simulink model "HW2_FSR_ES4"  (R2023b)
settings: Solver=FixedStepAuto  StartTime=0.0  StopTime=T  FixedStep=Ts  RelTol=1e-5
values from neighbouring files (symbols this model uses):
  k1 = 1    [HW2_FSR_ES4_Script.m]
  k2 = 2    [HW2_FSR_ES4_Script.m]
  k3 = 1    [HW2_FSR_ES4_Script.m]
  q_i = [10 1 pi\4]'    [HW2_FSR_ES4_Script.m]
  Ts = 0.01    [HW2_FSR_ES4_Script.m]
libraries: robotmobilelib x1
settings Model: Creator=emman  LastModifiedBy=emman

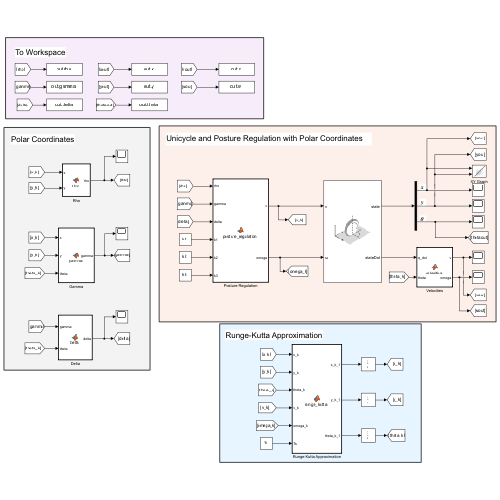
[thumbnail: Simulink's stored preview of the top-level diagram]
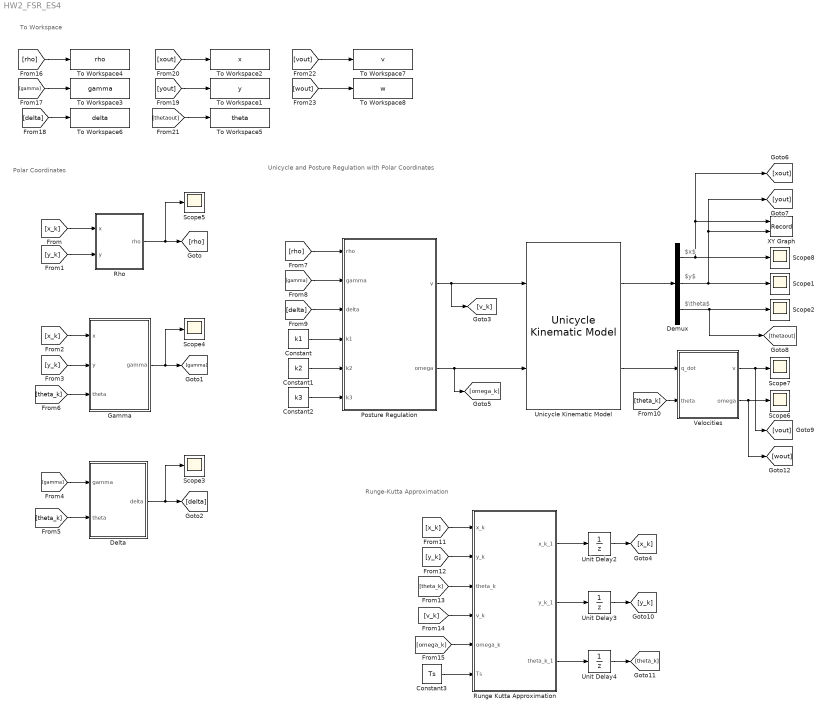
== system HW2_FSR_ES4 ==
  note: To Workspace
  note: Polar Coordinates
  note: Unicycle and Posture Regulation with Polar Coordinates
  note: $x$
  note: Runge-Kutta Approximation
  note: $y$
  note: $\theta$
  Constant : Constant  Value=k1
  Constant1 : Constant  Value=k2
  Constant2 : Constant  Value=k3
  Constant3 : Constant  Value=Ts
  Delta : MATLAB Function  TreatAsAtomicUnit=on
  Demux : Demux  Outputs=3
  Gamma : MATLAB Function  TreatAsAtomicUnit=on
  Posture Regulation : MATLAB Function  TreatAsAtomicUnit=on
  Rho : MATLAB Function  TreatAsAtomicUnit=on
  Runge Kutta Approximation : MATLAB Function  TreatAsAtomicUnit=on
  Scope{1..8} (8 alike) : Scope
  To Workspace1 : ToWorkspace  VariableName=y  SaveFormat=Timeseries  SampleTime=-1
  To Workspace2 : ToWorkspace  VariableName=x  SaveFormat=Timeseries  SampleTime=-1
  To Workspace3 : ToWorkspace  VariableName=gamma  SaveFormat=Timeseries  SampleTime=-1
  To Workspace4 : ToWorkspace  VariableName=rho  SaveFormat=Timeseries  SampleTime=-1
  To Workspace5 : ToWorkspace  VariableName=theta  SaveFormat=Timeseries  SampleTime=-1
  To Workspace6 : ToWorkspace  VariableName=delta  SaveFormat=Timeseries  SampleTime=-1
  To Workspace7 : ToWorkspace  VariableName=v  SaveFormat=Timeseries  SampleTime=-1
  To Workspace8 : ToWorkspace  VariableName=w  SaveFormat=Timeseries  SampleTime=-1
  Unicycle Kinematic Model : robotmobilelib/Unicycle Kinematic Model  VehicleInputs=Vehicle Speed & Heading Angular Velocity  WheelRadius=0.1  WheelSpeedRange=[-Inf Inf]  InitialState=q_i  SimulateUsing=Interpreted execution
  Unit Delay2 : UnitDelay  InitialCondition=q_i(1)  SampleTime=Ts  HasFrameUpgradeWarning=on
  Unit Delay3 : UnitDelay  InitialCondition=q_i(2)  SampleTime=Ts  HasFrameUpgradeWarning=on
  Unit Delay4 : UnitDelay  InitialCondition=q_i(3)  SampleTime=Ts  HasFrameUpgradeWarning=on
  Velocities : MATLAB Function  TreatAsAtomicUnit=on
  XY Graph : Record  FileSettingsInternal="{\"entries\":[{\"content\":{\"excelSettings\":{\"content\":{},\"type\":\"Streamout.ExcelSettings\"}},\"type\":\"Streamout.FileSettingStorage\",\"uuid\":\"\"}],\"packageUris\":[\"http:\\/\\/schema.mathworks.com\\/mf0\\/streamout_blocks\\/R2020a\"],\"version\":\"1.0\"}"  Layout=[1 1]  SignalsInternal="{\"entries\":[{\"content\":{\"signals\":[{\"content\":{\"blockPath\":[],\"dimensions\":[1],\"domain\":\"\",\"lineColor\":\"#a2142f\",\"plots\":[1],\"port\":1,\"sid\":[\"\"],\"signalID\":907,\"signalName\":\"Demux:1\"},\"type\":\"RecordBlkView.Signal\",\"uuid\":\"\"},{\"content\":{\"blockPath\":[],\"dimensions\":[1],\"domain\":\"\",\"lineColor\":\"#139fff\",\"plots\":[1],\"port\":2,\"sid\":[\"\"],\"signalID\":911,\"signalName\":\"Demux:2\"},\"type\":\"RecordBlkView.Signal\",\"uuid\":\"\"}]},\"type\":\"RecordBlkView.InputSignals\",\"uuid\":\"\"}],\"packageUris\":[\"http:\\/\\/schema.mathworks.com\\/mf0\\/streamout_blocks\\/R2020a\"],\"version\":\"1.0\"}"  VisualizationBindings="{\"xyplotplugin\":{\"info\":[{\"series\":[{\"bindingParametersList\":[{\"parameter\":\"X-Axis\",\"signalID\":907,\"signalName\":\"Demux:1\"},{\"parameter\":\"Y-Axis\",\"signalID\":911,\"signalName\":\"Demux:2\"}],\"seriesID\":55378}],\"subplotID\":1}]}}"  CompatibilityTag=XY
  wires:
  [x_k] -> Rho/1(x)
  [y_k] -> Rho/2(y)
  [x_k] -> Gamma/1(x)
  [y_k] -> Gamma/2(y)
  Delta/1(delta) -> Scope3/1, [delta]
  Gamma/1(gamma) -> Scope4/1, [gamma]
  Rho/1(rho) -> Scope5/1, [rho]
  [gamma] -> Delta/1(gamma)
  [theta_k] -> Delta/2(theta)
  [theta_k] -> Gamma/3(theta)
  Constant2/1 -> Posture Regulation/6(k3)
  Constant1/1 -> Posture Regulation/5(k2)
  Constant/1 -> Posture Regulation/4(k1)
  [delta] -> Posture Regulation/3(delta)
  [gamma] -> Posture Regulation/2(gamma)
  [rho] -> Posture Regulation/1(rho)
  Posture Regulation/2(omega) -> Unicycle Kinematic Model/2, [omega_k]
  Unicycle Kinematic Model/2 -> Velocities/1(q_dot)
  [theta_k] -> Velocities/2(theta)
  Velocities/1(v) -> [vout], Scope7/1
  Velocities/2(omega) -> [wout], Scope6/1
  Runge Kutta Approximation/1(x_k_1) -> Unit Delay2/1
  Runge Kutta Approximation/2(y_k_1) -> Unit Delay3/1
  Runge Kutta Approximation/3(theta_k_1) -> Unit Delay4/1
  Unit Delay2/1 -> [x_k]
  Unit Delay3/1 -> [y_k]
  Unit Delay4/1 -> [theta_k]
  [x_k] -> Runge Kutta Approximation/1(x_k)
  [theta_k] -> Runge Kutta Approximation/3(theta_k)
  [y_k] -> Runge Kutta Approximation/2(y_k)
  [v_k] -> Runge Kutta Approximation/4(v_k)
  [omega_k] -> Runge Kutta Approximation/5(omega_k)
  Constant3/1 -> Runge Kutta Approximation/6(Ts)
  Demux/1 -> Scope8/1, [xout], XY Graph/1
  Demux/2 -> [yout], XY Graph/2, Scope1/1
  Demux/3 -> [thetaout], Scope2/1
  Unicycle Kinematic Model/1 -> Demux/1
  Posture Regulation/1(v) -> Unicycle Kinematic Model/1, [v_k]
  [xout] -> To Workspace2/1
  [yout] -> To Workspace1/1
  [thetaout] -> To Workspace5/1
  [delta] -> To Workspace6/1
  [gamma] -> To Workspace3/1
  [rho] -> To Workspace4/1
  [vout] -> To Workspace7/1
  [wout] -> To Workspace8/1

== matlab function HW2_FSR_ES4/Gamma ==
  data: x input; gamma output; y input; theta input
function gamma = gamma(x, y, theta)

gamma = atan2(y,x) - theta + pi;

== matlab function HW2_FSR_ES4/Rho ==
  data: x input; rho output; y input
function rho = rho(x, y)

rho = sqrt(x^2 + y^2);

== matlab function HW2_FSR_ES4/Delta ==
  data: gamma input; delta output; theta input
function delta = delta(gamma, theta)

delta = gamma + theta;

== matlab function HW2_FSR_ES4/Posture Regulation ==
  data: rho input; v output; omega output; gamma input; delta input; k1 input; k2 input; k3 input
function [v,omega] = posture_regulation(rho, gamma, delta, k1, k2, k3)

v = k1*rho*cos(gamma);
omega = k2*gamma + k1*sin(gamma)*cos(gamma)*(1+k3*delta/gamma);

== matlab function HW2_FSR_ES4/Runge Kutta Approximation ==
  data: x_k input; x_k_1 output; y_k input; y_k_1 output; theta_k_1 output; theta_k input; v_k input; omega_k input; Ts input
function [x_k_1, y_k_1, theta_k_1] = runge_kutta(x_k, y_k, theta_k, v_k, omega_k, Ts)

x_k_1 = x_k + v_k*Ts*cos(theta_k + 1/2*omega_k*Ts);
y_k_1 = y_k + v_k*Ts*sin(theta_k + 1/2*omega_k*Ts);
theta_k_1 = theta_k + omega_k*Ts;

== matlab function HW2_FSR_ES4/Velocities ==
  data: q_dot input; v output; theta input; omega output
function [v, omega] = velocities(q_dot, theta)

v = q_dot(1)/cos(theta);
omega = q_dot(3);
